simulink model "Control_v8_PID_LLSat"  (R2023b)
settings: Solver=FixedStepAuto  StartTime=0.0  StopTime=t_sim  FixedStep=TimeStep  RelTol=1e-3
values from neighbouring files (symbols this model uses):
  MODE = 2    [main_SCA_v3.m]    (also in main_SCA_v3_alt.m; main_SCA_v4_LQR.m; main_SCA_v5.m = 1)
  Use_IGRF = 0    [main_SCA.m]    (also in main_SCA_v3.m; main_SCA_v3_alt.m; main_SCA_v4_LQR.m; main_SCA_v5.m = 1)
undefined symbols (not defined in the file or in its folder): att, B, date, deg, DipoleMod, DiscIntNeverNeededParam, LLSataero, orbit, rad, s, sat
libraries: vrlib x21, aerolibutil x17, dspmathops x15, aerolibconvert2 x14, sharedtransform x14, sharedutil x5, simulink x4, simulink_extras x2, dspstat3 x1, aerolibatmos2 x1, aerolibobsolete x1
(part 2 of 3)

== system Control_v8_PID_LLSat/Attitude Reference/Switch Case Action Subsystem1 ==
  Q_retro : Inport
  W_retro : Inport  Port=2
  Action Port : ActionPort  ActionPortLabel=case [ 5 ]:
  Out1 : Outport  VectorParamsAs1DForOutWhenUnconnected=off
  Out3 : Outport  Port=2  VectorParamsAs1DForOutWhenUnconnected=off
  wires:
  Q_retro/1 -> Out1/1
  W_retro/1 -> Out3/1

== system Control_v8_PID_LLSat/Attitude Reference/Switch Case Action Subsystem10 ==
  note: from I to SS
  Q_roll : Inport
  W_roll : Inport  Port=2
  Action Port : ActionPort  ActionPortLabel=case [ 10 ]:
  Out1 : Outport  VectorParamsAs1DForOutWhenUnconnected=off
  Out3 : Outport  Port=2  VectorParamsAs1DForOutWhenUnconnected=off
  wires:
  Q_roll/1 -> Out1/1
  W_roll/1 -> Out3/1

== system Control_v8_PID_LLSat/Attitude Reference/Switch Case Action Subsystem11 ==
  note: from I to SS
  Q_roll : Inport
  W_roll : Inport  Port=2
  Action Port : ActionPort  ActionPortLabel=case [ 11 ]:
  Out1 : Outport  VectorParamsAs1DForOutWhenUnconnected=off
  Out3 : Outport  Port=2  VectorParamsAs1DForOutWhenUnconnected=off
  wires:
  Q_roll/1 -> Out1/1
  W_roll/1 -> Out3/1

== system Control_v8_PID_LLSat/Attitude Reference/Switch Case Action Subsystem2 ==
  note: q from I to O + rotation
  Q_drag : Inport
  W_drag : Inport  Port=2
  Action Port : ActionPort  ActionPortLabel=case [ 4 ]:
  Out1 : Outport  VectorParamsAs1DForOutWhenUnconnected=off
  W : Outport  Port=2
  wires:
  Q_drag/1 -> Out1/1
  W_drag/1 -> W/1

== system Control_v8_PID_LLSat/Attitude Reference/Switch Case Action Subsystem3 ==
  Q_sun_sun : Inport
  W_sun_sun : Inport  Port=2
  Action Port : ActionPort  ActionPortLabel=case [ 3 ]:
  Out1 : Outport  VectorParamsAs1DForOutWhenUnconnected=off
  Out3 : Outport  Port=2  VectorParamsAs1DForOutWhenUnconnected=off
  wires:
  Q_sun_sun/1 -> Out1/1
  W_sun_sun/1 -> Out3/1

== system Control_v8_PID_LLSat/Attitude Reference/Switch Case Action Subsystem4 ==
  Q_sun_aero : Inport
  W_sun_aero : Inport  Port=2
  Action Port : ActionPort  ActionPortLabel=case [ 2 ]:
  Out1 : Outport  VectorParamsAs1DForOutWhenUnconnected=off
  Out3 : Outport  Port=2  VectorParamsAs1DForOutWhenUnconnected=off
  wires:
  Q_sun_aero/1 -> Out1/1
  W_sun_aero/1 -> Out3/1

== system Control_v8_PID_LLSat/Attitude Reference/Switch Case Action Subsystem5 ==
  In1 : Inport
  W_orbit : Inport  Port=2
  Action Port : ActionPort  ActionPortLabel=case [ 1 ]:
  Out1 : Outport  VectorParamsAs1DForOutWhenUnconnected=off
  Out3 : Outport  Port=2  VectorParamsAs1DForOutWhenUnconnected=off
  wires:
  In1/1 -> Out1/1
  W_orbit/1 -> Out3/1

== system Control_v8_PID_LLSat/Attitude Reference/Switch Case Action Subsystem6 ==
  In1 : Inport
  In2 : Inport  Port=2
  Action Port : ActionPort  ActionPortLabel=case [ 7 ]:
  Derivative : Derivative
  Matrix Multiply : Product  Multiplication=Matrix(*)
  Quaternions to Direction Cosine Matrix : sharedtransform/Quaternions to  Direction Cosine Matrix  aMode=aMode
  Transpose : Math  Operator=transpose
  Transpose1 : Math  Operator=transpose
  gets vector from Skew Matrix : MATLABFcn  MATLABFcn=vec_from_skew
  Out1 : Outport  VectorParamsAs1DForOutWhenUnconnected=off
  W_custom : Outport  Port=2
  wires:
  In1/1 -> Out1/1
  In2/1 -> Quaternions to Direction Cosine Matrix/1
  Quaternions to Direction Cosine Matrix/1 -> Transpose1/1
  Matrix Multiply/1 -> gets vector from Skew Matrix/1
  Transpose/1 -> Derivative/1
  gets vector from Skew Matrix/1 -> W_custom/1
  Derivative/1 -> Matrix Multiply/1
  Transpose1/1 -> Transpose/1, Matrix Multiply/2

== system Control_v8_PID_LLSat/Attitude Reference/Switch Case Action Subsystem7 ==
  In1 : Inport
  In2 : Inport  Port=2
  Action Port : ActionPort  ActionPortLabel=case [ 6 ]:
  Out1 : Outport  VectorParamsAs1DForOutWhenUnconnected=off
  Out2 : Outport  Port=2  VectorParamsAs1DForOutWhenUnconnected=off
  wires:
  In1/1 -> Out1/1
  In2/1 -> Out2/1

== system Control_v8_PID_LLSat/Attitude Reference/Switch Case Action Subsystem8 ==
  Q_retro : Inport
  W_retro : Inport  Port=2
  Action Port : ActionPort  ActionPortLabel=case [ 8 ]:
  Out1 : Outport  VectorParamsAs1DForOutWhenUnconnected=off
  Out3 : Outport  Port=2  VectorParamsAs1DForOutWhenUnconnected=off
  wires:
  Q_retro/1 -> Out1/1
  W_retro/1 -> Out3/1

== system Control_v8_PID_LLSat/Attitude Reference/Switch Case Action Subsystem9 ==
  note: q from I to O + rotation
  Q_rot : Inport
  W_rot : Inport  Port=2
  Action Port : ActionPort  ActionPortLabel=case [ 9 ]:
  Out1 : Outport  VectorParamsAs1DForOutWhenUnconnected=off
  W : Outport  Port=2
  wires:
  Q_rot/1 -> Out1/1
  W_rot/1 -> W/1

== system Control_v8_PID_LLSat/Attitude Reference/q_drag ==
  note: x in BRF is aligned with the zenith direction
      | z in BRF (solar panels) is aligned in the direction of velocity
  note: DCM from Drag to Inertial
  note: q from D to I
  note: q from I to D
  note: To get angular velocity from Rotation matrix:
      | https://en.wikipedia.org/wiki/Angular_velocity#Angular_velocity_tensor
      | W= dA/dt * A'
      | $W=\frac{dA}{dt} {\dot} A'=\frac{dA}{dt} {\dot} A^{T}$
  <XYZ_ECI> : Inport
  <VxVyVz_ECI> : Inport  Port=2
  3x3 Cross Product : sharedutil/3x3 Cross Product  aMode=aMode
  Derivative : Derivative
  Direction Cosine Matrix to Quaternions : sharedtransform/Direction Cosine Matrix  to Quaternions  aMode=0  action=None  tolerance=eps(2)
  Gain : Gain
  Gain1 : Gain
  Matrix Multiply : Product  Multiplication=Matrix(*)
  Normalization : dspmathops/Normalization  NormType=2-norm  Bias=1e-10  NormOver=Each column  Dimension=1  roundingMode=Floor  overflowMode=off  accumDataTypeStr=Inherit: Same as product output  accumLastDataTypeStr=Inherit: Same as product output  outputDataTypeStr=Inherit: Same as product output  outputMin=[]  outputMax=[]  outputLastDataTypeStr=Inherit: Same as product output
  Normalization1 : dspmathops/Normalization  NormType=2-norm  Bias=1e-10  NormOver=Each column  Dimension=1  roundingMode=Floor  overflowMode=off  accumDataTypeStr=Inherit: Same as product output  accumLastDataTypeStr=Inherit: Same as product output  outputDataTypeStr=Inherit: Same as product output  outputMin=[]  outputMax=[]  outputLastDataTypeStr=Inherit: Same as product output
  Quaternion Inverse : aerolibutil/Quaternion Inverse
  Reshape : Reshape  OutputDimensionality=Column vector (2-D)
  Reshape1 : Reshape  OutputDimensionality=Column vector (2-D)
  Reshape2 : Reshape  OutputDimensionality=Column vector (2-D)
  Reshape3 : Reshape  OutputDimensionality=Customize  OutputDimensions=[3,3]
  Transpose : Math  Operator=transpose
  Vector Concatenate : Concatenate  NumInputs=3  Mode=Multidimensional array  ConcatenateDimension=2
  gets vector from Skew Matrix : MATLABFcn  MATLABFcn=vec_from_skew
  Q_drag : Outport  VectorParamsAs1DForOutWhenUnconnected=off
  W_drag : Outport  Port=2
  wires:
  Normalization/1 -> Reshape/1
  Normalization1/1 -> Reshape1/1
  <VxVyVz_ECI>/1 -> Normalization1/1
  Reshape1/1 -> Vector Concatenate/3, 3x3 Cross Product/1
  <XYZ_ECI>/1 -> Normalization/1
  Reshape/1 -> Gain/1
  Gain/1 -> Vector Concatenate/1, 3x3 Cross Product/2
  Direction Cosine Matrix to Quaternions/1 -> Quaternion Inverse/1
  3x3 Cross Product/1 -> Gain1/1
  Gain1/1 -> Reshape2/1
  Quaternion Inverse/1 -> Q_drag/1
  Vector Concatenate/1 -> Reshape3/1, Direction Cosine Matrix to Quaternions/1
  gets vector from Skew Matrix/1 -> W_drag/1
  Matrix Multiply/1 -> gets vector from Skew Matrix/1
  Transpose/1 -> Derivative/1
  Derivative/1 -> Matrix Multiply/1
  Reshape2/1 -> Vector Concatenate/2
  Reshape3/1 -> Matrix Multiply/2, Transpose/1

== system Control_v8_PID_LLSat/Attitude Reference/q_orbital ==
  note: DCM from Orbital to Inertial
  note: q from O to I
  note: q from I to O
  note: To get angular velocity from Rotation matrix:
      | https://en.wikipedia.org/wiki/Angular_velocity#Angular_velocity_tensor
      | W= dA/dt * A'
      | $W=\frac{dA}{dt} {\dot} A'=\frac{dA}{dt} {\dot} A^{T}$
  <XYZ_ECI> : Inport
  <VxVyVz_ECI> : Inport  Port=2
  3x3 Cross Product : sharedutil/3x3 Cross Product  aMode=aMode
  Derivative : Derivative
  Direction Cosine Matrix to Quaternions : sharedtransform/Direction Cosine Matrix  to Quaternions  aMode=0  action=None  tolerance=eps(2)
  Gain : Gain
  Gain1 : Gain  Gain=-1
  Matrix Multiply : Product  Multiplication=Matrix(*)
  Normalization : dspmathops/Normalization  NormType=2-norm  Bias=1e-10  NormOver=Each column  Dimension=1  roundingMode=Floor  overflowMode=off  accumDataTypeStr=Inherit: Same as product output  accumLastDataTypeStr=Inherit: Same as product output  outputDataTypeStr=Inherit: Same as product output  outputMin=[]  outputMax=[]  outputLastDataTypeStr=Inherit: Same as product output
  Normalization1 : dspmathops/Normalization  NormType=2-norm  Bias=1e-10  NormOver=Each column  Dimension=1  roundingMode=Floor  overflowMode=off  accumDataTypeStr=Inherit: Same as product output  accumLastDataTypeStr=Inherit: Same as product output  outputDataTypeStr=Inherit: Same as product output  outputMin=[]  outputMax=[]  outputLastDataTypeStr=Inherit: Same as product output
  Quaternion Inverse : aerolibutil/Quaternion Inverse
  Reshape : Reshape  OutputDimensionality=Column vector (2-D)
  Reshape1 : Reshape  OutputDimensionality=Column vector (2-D)
  Reshape2 : Reshape  OutputDimensionality=Column vector (2-D)
  Reshape3 : Reshape  OutputDimensionality=Customize  OutputDimensions=[3,3]
  Transpose : Math  Operator=transpose
  Vector Concatenate : Concatenate  NumInputs=3  Mode=Multidimensional array  ConcatenateDimension=2
  gets vector from Skew Matrix : MATLABFcn  MATLABFcn=vec_from_skew
  Q_orbit : Outport  VectorParamsAs1DForOutWhenUnconnected=off
  W_orbit : Outport  Port=2
  wires:
  Normalization/1 -> Reshape/1
  Normalization1/1 -> Reshape1/1
  <VxVyVz_ECI>/1 -> Normalization1/1
  Reshape1/1 -> 3x3 Cross Product/1, Vector Concatenate/1
  <XYZ_ECI>/1 -> Normalization/1
  Reshape/1 -> Gain/1
  Gain/1 -> 3x3 Cross Product/2, Vector Concatenate/3
  Direction Cosine Matrix to Quaternions/1 -> Quaternion Inverse/1
  3x3 Cross Product/1 -> Gain1/1
  Gain1/1 -> Reshape2/1
  Quaternion Inverse/1 -> Q_orbit/1
  Vector Concatenate/1 -> Reshape3/1, Direction Cosine Matrix to Quaternions/1
  gets vector from Skew Matrix/1 -> W_orbit/1
  Matrix Multiply/1 -> gets vector from Skew Matrix/1
  Transpose/1 -> Derivative/1
  Derivative/1 -> Matrix Multiply/1
  Reshape2/1 -> Vector Concatenate/2
  Reshape3/1 -> Matrix Multiply/2, Transpose/1

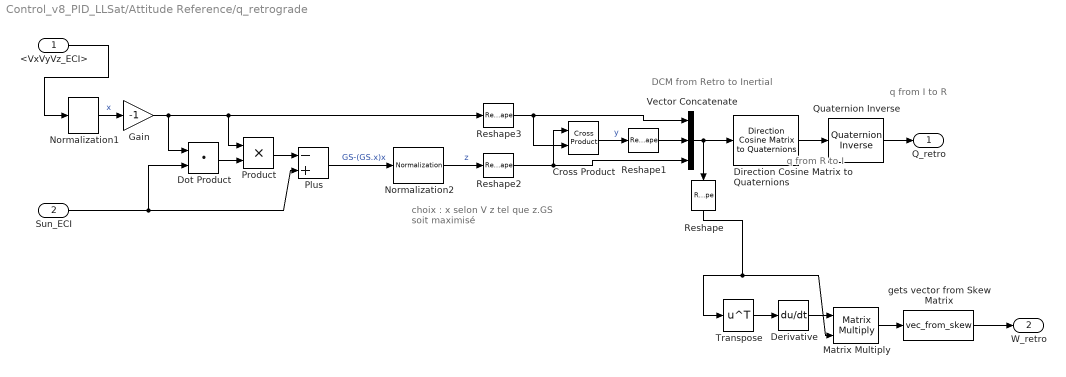
== system Control_v8_PID_LLSat/Attitude Reference/q_retrograde ==
  note: q from I to R
  note: q from R to I
  note: DCM from Retro to Inertial
  note: choix :
      | x selon V
      | z tel que z.GS soit maximisé
  <VxVyVz_ECI> : Inport
  Sun_ECI : Inport  Port=2
  Cross Product : vrlib/Utilities/Cross Product
  Derivative : Derivative
  Direction Cosine Matrix to Quaternions : sharedtransform/Direction Cosine Matrix  to Quaternions  aMode=0  action=None  tolerance=eps(2)
  Dot Product : DotProduct  OutDataTypeStr=Inherit: Inherit via internal rule
  Gain : Gain  Gain=-1
  Matrix Multiply : Product  Multiplication=Matrix(*)
  Normalization1 : dspmathops/Normalization  NormType=2-norm  Bias=1e-10  NormOver=Each column  Dimension=1  roundingMode=Floor  overflowMode=off  accumDataTypeStr=Inherit: Same as product output  accumLastDataTypeStr=Inherit: Same as product output  outputDataTypeStr=Inherit: Same as product output  outputMin=[]  outputMax=[]  outputLastDataTypeStr=Inherit: Same as product output
  Normalization2 : dspmathops/Normalization  NormType=2-norm  Bias=1e-10  NormOver=Each column  Dimension=1  roundingMode=Floor  overflowMode=off  accumDataTypeStr=Inherit: Same as product output  accumLastDataTypeStr=Inherit: Same as product output  outputDataTypeStr=Inherit: Same as product output  outputMin=[]  outputMax=[]  outputLastDataTypeStr=Inherit: Same as product output
  Plus : Sum  Inputs=-+
  Product : Product
  Quaternion Inverse : aerolibutil/Quaternion Inverse
  Reshape : Reshape  OutputDimensionality=Customize  OutputDimensions=[3,3]
  Reshape1 : Reshape  OutputDimensionality=Column vector (2-D)
  Reshape2 : Reshape  OutputDimensionality=Column vector (2-D)
  Reshape3 : Reshape  OutputDimensionality=Column vector (2-D)
  Transpose : Math  Operator=transpose
  Vector Concatenate : Concatenate  NumInputs=3  Mode=Multidimensional array  ConcatenateDimension=2
  gets vector from Skew Matrix : MATLABFcn  MATLABFcn=vec_from_skew
  Q_retro : Outport  VectorParamsAs1DForOutWhenUnconnected=off
  W_retro : Outport  Port=2
  wires:
  Quaternion Inverse/1 -> Q_retro/1
  Reshape2/1 -> Vector Concatenate/3, Cross Product/1
  Reshape3/1 -> Vector Concatenate/1, Cross Product/2
  Product/1 -> Plus/1
  Dot Product/1 -> Product/2
  Cross Product/1 -> Reshape1/1  "y"
  Normalization2/1 -> Reshape2/1  "z"
  Plus/1 -> Normalization2/1  "GS-(GS.x)x"
  Sun_ECI/1 -> Dot Product/2, Plus/2
  Direction Cosine Matrix to Quaternions/1 -> Quaternion Inverse/1
  Normalization1/1 -> Gain/1  "x"
  <VxVyVz_ECI>/1 -> Normalization1/1
  Reshape1/1 -> Vector Concatenate/2
  Gain/1 -> Dot Product/1, Product/1, Reshape3/1
  Vector Concatenate/1 -> Direction Cosine Matrix to Quaternions/1, Reshape/1
  gets vector from Skew Matrix/1 -> W_retro/1
  Matrix Multiply/1 -> gets vector from Skew Matrix/1
  Derivative/1 -> Matrix Multiply/1
  Transpose/1 -> Derivative/1
  Reshape/1 -> Transpose/1, Matrix Multiply/2

== system Control_v8_PID_LLSat/Attitude Reference/q_sun_aero ==
  note: q from I to S
  note: q from S to I
  note: DCM from Sun-aero to Inertial
  note: choix :
      | x selon V
      | z tel que z.GS soit maximisé
  Sun_ECI : Inport
  <VxVyVz_ECI> : Inport  Port=2
  Cross Product : vrlib/Utilities/Cross Product
  Derivative : Derivative
  Direction Cosine Matrix to Quaternions : sharedtransform/Direction Cosine Matrix  to Quaternions  aMode=0  action=None  tolerance=eps(2)
  Dot Product : DotProduct  OutDataTypeStr=Inherit: Inherit via internal rule
  Matrix Multiply : Product  Multiplication=Matrix(*)
  Normalization1 : dspmathops/Normalization  NormType=2-norm  Bias=1e-10  NormOver=Each column  Dimension=1  roundingMode=Floor  overflowMode=off  accumDataTypeStr=Inherit: Same as product output  accumLastDataTypeStr=Inherit: Same as product output  outputDataTypeStr=Inherit: Same as product output  outputMin=[]  outputMax=[]  outputLastDataTypeStr=Inherit: Same as product output
  Normalization2 : dspmathops/Normalization  NormType=2-norm  Bias=1e-10  NormOver=Each column  Dimension=1  roundingMode=Floor  overflowMode=off  accumDataTypeStr=Inherit: Same as product output  accumLastDataTypeStr=Inherit: Same as product output  outputDataTypeStr=Inherit: Same as product output  outputMin=[]  outputMax=[]  outputLastDataTypeStr=Inherit: Same as product output
  Plus : Sum  Inputs=-+
  Product : Product
  Quaternion Inverse : aerolibutil/Quaternion Inverse
  Reshape : Reshape  OutputDimensionality=Customize  OutputDimensions=[3,3]
  Reshape1 : Reshape  OutputDimensionality=Column vector (2-D)
  Reshape2 : Reshape  OutputDimensionality=Column vector (2-D)
  Reshape3 : Reshape  OutputDimensionality=Column vector (2-D)
  Transpose : Math  Operator=transpose
  Vector Concatenate : Concatenate  NumInputs=3  Mode=Multidimensional array  ConcatenateDimension=2
  gets vector from Skew Matrix : MATLABFcn  MATLABFcn=vec_from_skew
  Q_sun_aero : Outport  VectorParamsAs1DForOutWhenUnconnected=off
  W_sun_aero : Outport  Port=2
  wires:
  Quaternion Inverse/1 -> Q_sun_aero/1
  Reshape2/1 -> Vector Concatenate/3, Cross Product/1
  Reshape3/1 -> Vector Concatenate/1, Cross Product/2
  Product/1 -> Plus/1
  Dot Product/1 -> Product/2
  Cross Product/1 -> Reshape1/1  "y"
  Normalization2/1 -> Reshape2/1  "z"
  Plus/1 -> Normalization2/1  "GS-(GS.x)x"
  Sun_ECI/1 -> Dot Product/2, Plus/2
  Direction Cosine Matrix to Quaternions/1 -> Quaternion Inverse/1
  Normalization1/1 -> Dot Product/1, Product/1, Reshape3/1  "x"
  <VxVyVz_ECI>/1 -> Normalization1/1
  Reshape1/1 -> Vector Concatenate/2
  Transpose/1 -> Derivative/1
  Matrix Multiply/1 -> gets vector from Skew Matrix/1
  Derivative/1 -> Matrix Multiply/1
  Vector Concatenate/1 -> Direction Cosine Matrix to Quaternions/1, Reshape/1
  gets vector from Skew Matrix/1 -> W_sun_aero/1
  Reshape/1 -> Transpose/1, Matrix Multiply/2

== system Control_v8_PID_LLSat/Attitude Reference/q_sun_aero_rotation_x_pi//1 ==
  Q_sun_aero : Inport
  Q_sun_sun : Inport  Port=2
  In3 : Inport  Port=3
  Quaternion Interpolation : QuatInterp
  Quaternion Normalize : sharedutil/Quaternion Normalize  aMode=aMode
  Quaternion Normalize1 : sharedutil/Quaternion Normalize  aMode=aMode
  Q_slerp : Outport  VectorParamsAs1DForOutWhenUnconnected=off
  wires:
  Quaternion Interpolation/1 -> Q_slerp/1
  Q_sun_sun/1 -> Quaternion Normalize1/1
  Q_sun_aero/1 -> Quaternion Normalize/1
  In3/1 -> Quaternion Interpolation/3
  Quaternion Normalize/1 -> Quaternion Interpolation/1
  Quaternion Normalize1/1 -> Quaternion Interpolation/2

== system Control_v8_PID_LLSat/Attitude Reference/q_sun_aero_rotation_x_pi//4 ==
  Constant : Constant  Value=[1;0;0]
  Product : Product
  Reshape1 : Reshape  OutputDimensionality=Column vector (2-D)
  Vector Concatenate1 : Concatenate  Mode=Multidimensional array
  cos pi/2 : Constant  Value=[cos(-att.angle_roll/2)]
  sin pi/4 : Constant  Value=sin(-att.angle_roll/2)
  Q_rot : Outport  VectorParamsAs1DForOutWhenUnconnected=off
  wires:
  cos pi/2/1 -> Vector Concatenate1/1
  Vector Concatenate1/1 -> Q_rot/1
  sin pi/4/1 -> Product/2
  Product/1 -> Reshape1/1
  Reshape1/1 -> Vector Concatenate1/2
  Constant/1 -> Product/1  "x"

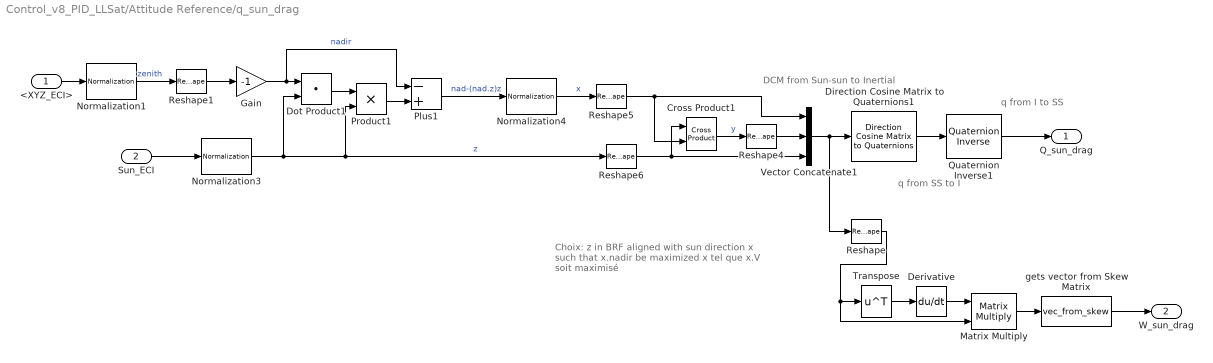
== system Control_v8_PID_LLSat/Attitude Reference/q_sun_drag ==
  note: Choix:
      | z in BRF aligned with sun direction
      | x such that x.nadir be maximized
      | x tel que x.V soit maximisé
  note: DCM from Sun-sun to Inertial
  note: q from I to SS
  note: q from SS to I
  <XYZ_ECI> : Inport
  Sun_ECI : Inport  Port=2
  Cross Product1 : vrlib/Utilities/Cross Product
  Derivative : Derivative
  Direction Cosine Matrix to Quaternions1 : sharedtransform/Direction Cosine Matrix  to Quaternions  aMode=0  action=None  tolerance=eps(2)
  Dot Product1 : DotProduct  OutDataTypeStr=Inherit: Inherit via internal rule
  Gain : Gain  Gain=-1
  Matrix Multiply : Product  Multiplication=Matrix(*)
  Normalization1 : dspmathops/Normalization  NormType=2-norm  Bias=1e-10  NormOver=Each column  Dimension=1  roundingMode=Floor  overflowMode=off  accumDataTypeStr=Inherit: Same as product output  accumLastDataTypeStr=Inherit: Same as product output  outputDataTypeStr=Inherit: Same as product output  outputMin=[]  outputMax=[]  outputLastDataTypeStr=Inherit: Same as product output
  Normalization3 : dspmathops/Normalization  NormType=2-norm  Bias=1e-10  NormOver=Each column  Dimension=1  roundingMode=Floor  overflowMode=off  accumDataTypeStr=Inherit: Same as product output  accumLastDataTypeStr=Inherit: Same as product output  outputDataTypeStr=Inherit: Same as product output  outputMin=[]  outputMax=[]  outputLastDataTypeStr=Inherit: Same as product output
  Normalization4 : dspmathops/Normalization  NormType=2-norm  Bias=1e-10  NormOver=Each column  Dimension=1  roundingMode=Floor  overflowMode=off  accumDataTypeStr=Inherit: Same as product output  accumLastDataTypeStr=Inherit: Same as product output  outputDataTypeStr=Inherit: Same as product output  outputMin=[]  outputMax=[]  outputLastDataTypeStr=Inherit: Same as product output
  Plus1 : Sum  Inputs=-+
  Product1 : Product
  Quaternion Inverse1 : aerolibutil/Quaternion Inverse
  Reshape : Reshape  OutputDimensionality=Customize  OutputDimensions=[3,3]
  Reshape{1,4..6} (4 alike) : Reshape  OutputDimensionality=Column vector (2-D)
  Transpose : Math  Operator=transpose
  Vector Concatenate1 : Concatenate  NumInputs=3  Mode=Multidimensional array  ConcatenateDimension=2
  gets vector from Skew Matrix : MATLABFcn  MATLABFcn=vec_from_skew
  Q_sun_drag : Outport  VectorParamsAs1DForOutWhenUnconnected=off
  W_sun_drag : Outport  Port=2
  wires:
  Direction Cosine Matrix to Quaternions1/1 -> Quaternion Inverse1/1
  Reshape4/1 -> Vector Concatenate1/2
  Dot Product1/1 -> Product1/1
  Sun_ECI/1 -> Normalization3/1
  Quaternion Inverse1/1 -> Q_sun_drag/1
  Reshape1/1 -> Gain/1
  Plus1/1 -> Normalization4/1  "nad-(nad.z)z"
  Reshape6/1 -> Cross Product1/1, Vector Concatenate1/3
  Normalization3/1 -> Dot Product1/2, Product1/2, Reshape6/1  "z"
  Reshape5/1 -> Cross Product1/2, Vector Concatenate1/1
  Cross Product1/1 -> Reshape4/1  "y"
  Normalization4/1 -> Reshape5/1  "x"
  Product1/1 -> Plus1/2
  Reshape/1 -> Matrix Multiply/2, Transpose/1
  Derivative/1 -> Matrix Multiply/1
  Transpose/1 -> Derivative/1
  Matrix Multiply/1 -> gets vector from Skew Matrix/1
  gets vector from Skew Matrix/1 -> W_sun_drag/1
  Vector Concatenate1/1 -> Direction Cosine Matrix to Quaternions1/1, Reshape/1
  <XYZ_ECI>/1 -> Normalization1/1
  Normalization1/1 -> Reshape1/1  "zenith"
  Gain/1 -> Dot Product1/1, Plus1/1  "nadir"

== system Control_v8_PID_LLSat/Attitude Reference/q_sun_sun ==
  note: Choix:
      | z selon GS
      | x tel que x.V soit maximisé
  note: DCM from Sun-sun to Inertial
  note: q from I to SS
  note: q from SS to I
  <VxVyVz_ECI> : Inport
  Sun_ECI : Inport  Port=2
  Cross Product1 : vrlib/Utilities/Cross Product
  Derivative : Derivative
  Direction Cosine Matrix to Quaternions1 : sharedtransform/Direction Cosine Matrix  to Quaternions  aMode=0  action=None  tolerance=eps(2)
  Dot Product1 : DotProduct  OutDataTypeStr=Inherit: Inherit via internal rule
  Matrix Multiply : Product  Multiplication=Matrix(*)
  Normalization3 : dspmathops/Normalization  NormType=2-norm  Bias=1e-10  NormOver=Each column  Dimension=1  roundingMode=Floor  overflowMode=off  accumDataTypeStr=Inherit: Same as product output  accumLastDataTypeStr=Inherit: Same as product output  outputDataTypeStr=Inherit: Same as product output  outputMin=[]  outputMax=[]  outputLastDataTypeStr=Inherit: Same as product output
  Normalization4 : dspmathops/Normalization  NormType=2-norm  Bias=1e-10  NormOver=Each column  Dimension=1  roundingMode=Floor  overflowMode=off  accumDataTypeStr=Inherit: Same as product output  accumLastDataTypeStr=Inherit: Same as product output  outputDataTypeStr=Inherit: Same as product output  outputMin=[]  outputMax=[]  outputLastDataTypeStr=Inherit: Same as product output
  Plus1 : Sum  Inputs=-+
  Product1 : Product
  Quaternion Inverse1 : aerolibutil/Quaternion Inverse
  Reshape : Reshape  OutputDimensionality=Customize  OutputDimensions=[3,3]
  Reshape4 : Reshape  OutputDimensionality=Column vector (2-D)
  Reshape5 : Reshape  OutputDimensionality=Column vector (2-D)
  Reshape6 : Reshape  OutputDimensionality=Column vector (2-D)
  Transpose : Math  Operator=transpose
  Vector Concatenate1 : Concatenate  NumInputs=3  Mode=Multidimensional array  ConcatenateDimension=2
  gets vector from Skew Matrix : MATLABFcn  MATLABFcn=vec_from_skew
  Q_sun_sun : Outport  VectorParamsAs1DForOutWhenUnconnected=off
  W_sun_sun : Outport  Port=2
  wires:
  Direction Cosine Matrix to Quaternions1/1 -> Quaternion Inverse1/1
  Reshape4/1 -> Vector Concatenate1/2
  Dot Product1/1 -> Product1/1
  Sun_ECI/1 -> Normalization3/1
  Quaternion Inverse1/1 -> Q_sun_sun/1
  <VxVyVz_ECI>/1 -> Dot Product1/1, Plus1/1
  Plus1/1 -> Normalization4/1  "V-(V.z)z"
  Reshape6/1 -> Cross Product1/1, Vector Concatenate1/3
  Normalization3/1 -> Dot Product1/2, Product1/2, Reshape6/1  "z"
  Reshape5/1 -> Cross Product1/2, Vector Concatenate1/1
  Cross Product1/1 -> Reshape4/1  "y"
  Normalization4/1 -> Reshape5/1  "x"
  Product1/1 -> Plus1/2
  Reshape/1 -> Matrix Multiply/2, Transpose/1
  Derivative/1 -> Matrix Multiply/1
  Transpose/1 -> Derivative/1
  Matrix Multiply/1 -> gets vector from Skew Matrix/1
  gets vector from Skew Matrix/1 -> W_sun_sun/1
  Vector Concatenate1/1 -> Direction Cosine Matrix to Quaternions1/1, Reshape/1

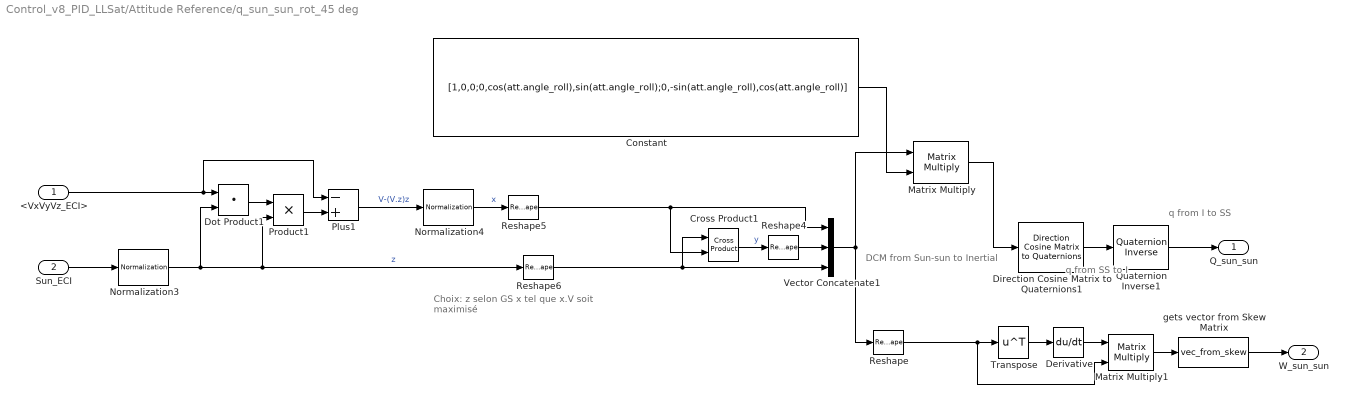
== system Control_v8_PID_LLSat/Attitude Reference/q_sun_sun_rot_45 deg ==
  note: Choix:
      | z selon GS
      | x tel que x.V soit maximisé
  note: DCM from Sun-sun to Inertial
  note: q from I to SS
  note: q from SS to I
  <VxVyVz_ECI> : Inport
  Sun_ECI : Inport  Port=2
  Constant : Constant  Value=[1,0,0;0,cos(att.angle_roll),sin(att.angle_roll);0,-sin(att.angle_roll),cos(att.angle_roll)]
  Cross Product1 : vrlib/Utilities/Cross Product
  Derivative : Derivative
  Direction Cosine Matrix to Quaternions1 : sharedtransform/Direction Cosine Matrix  to Quaternions  aMode=0  action=None  tolerance=eps(2)
  Dot Product1 : DotProduct  OutDataTypeStr=Inherit: Inherit via internal rule
  Matrix Multiply : Product  Multiplication=Matrix(*)
  Matrix Multiply1 : Product  Multiplication=Matrix(*)
  Normalization3 : dspmathops/Normalization  NormType=2-norm  Bias=1e-10  NormOver=Each column  Dimension=1  roundingMode=Floor  overflowMode=off  accumDataTypeStr=Inherit: Same as product output  accumLastDataTypeStr=Inherit: Same as product output  outputDataTypeStr=Inherit: Same as product output  outputMin=[]  outputMax=[]  outputLastDataTypeStr=Inherit: Same as product output
  Normalization4 : dspmathops/Normalization  NormType=2-norm  Bias=1e-10  NormOver=Each column  Dimension=1  roundingMode=Floor  overflowMode=off  accumDataTypeStr=Inherit: Same as product output  accumLastDataTypeStr=Inherit: Same as product output  outputDataTypeStr=Inherit: Same as product output  outputMin=[]  outputMax=[]  outputLastDataTypeStr=Inherit: Same as product output
  Plus1 : Sum  Inputs=-+
  Product1 : Product
  Quaternion Inverse1 : aerolibutil/Quaternion Inverse
  Reshape : Reshape  OutputDimensionality=Customize  OutputDimensions=[3,3]
  Reshape4 : Reshape  OutputDimensionality=Column vector (2-D)
  Reshape5 : Reshape  OutputDimensionality=Column vector (2-D)
  Reshape6 : Reshape  OutputDimensionality=Column vector (2-D)
  Transpose : Math  Operator=transpose
  Vector Concatenate1 : Concatenate  NumInputs=3  Mode=Multidimensional array  ConcatenateDimension=2
  gets vector from Skew Matrix : MATLABFcn  MATLABFcn=vec_from_skew
  Q_sun_sun : Outport  VectorParamsAs1DForOutWhenUnconnected=off
  W_sun_sun : Outport  Port=2
  wires:
  Reshape4/1 -> Vector Concatenate1/2
  Dot Product1/1 -> Product1/1
  Sun_ECI/1 -> Normalization3/1
  Quaternion Inverse1/1 -> Q_sun_sun/1
  <VxVyVz_ECI>/1 -> Dot Product1/1, Plus1/1
  Plus1/1 -> Normalization4/1  "V-(V.z)z"
  Reshape6/1 -> Cross Product1/1, Vector Concatenate1/3
  Normalization3/1 -> Dot Product1/2, Product1/2, Reshape6/1  "z"
  Reshape5/1 -> Cross Product1/2, Vector Concatenate1/1
  Cross Product1/1 -> Reshape4/1  "y"
  Normalization4/1 -> Reshape5/1  "x"
  Product1/1 -> Plus1/2
  Direction Cosine Matrix to Quaternions1/1 -> Quaternion Inverse1/1
  Constant/1 -> Matrix Multiply/2
  Vector Concatenate1/1 -> Matrix Multiply/1, Reshape/1
  Matrix Multiply/1 -> Direction Cosine Matrix to Quaternions1/1
  Transpose/1 -> Derivative/1
  gets vector from Skew Matrix/1 -> W_sun_sun/1
  Reshape/1 -> Matrix Multiply1/2, Transpose/1
  Derivative/1 -> Matrix Multiply1/1
  Matrix Multiply1/1 -> gets vector from Skew Matrix/1

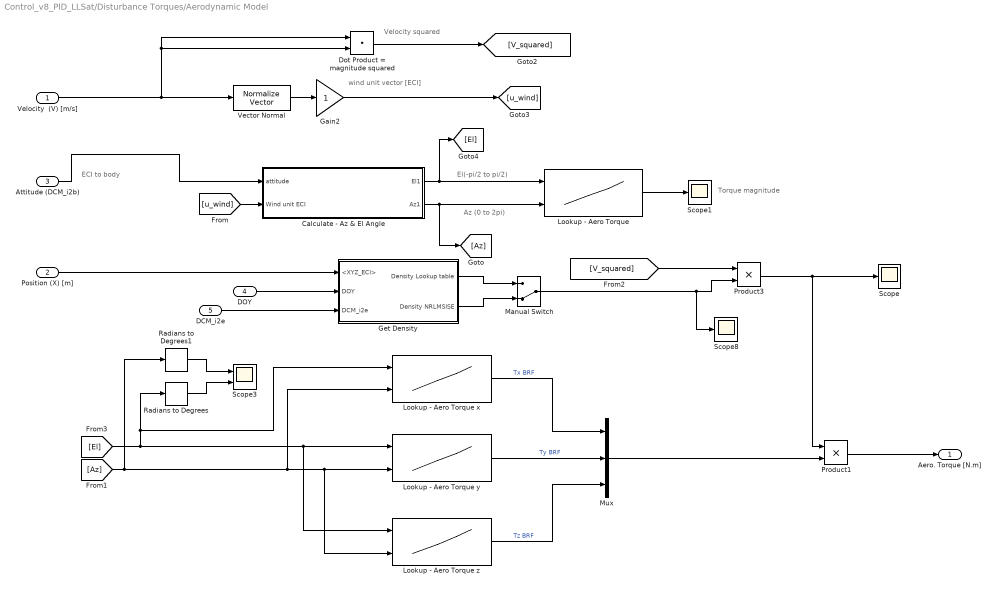
== system Control_v8_PID_LLSat/Disturbance Torques/Aerodynamic Model ==
  note: Az (0 to 2pi)
  note: wind unit vector [ECI]
  note: Torque magnitude
  note: ECI to body
  note: Velocity squared
  note: El(-pi/2 to pi/2)
  Velocity  (V) [m/s] : Inport
  Position (X) [m] : Inport  Port=2
  Attitude (DCM_i2b) : Inport  Port=3
  DOY : Inport  Port=4
  DCM_i2e : Inport  Port=5
  Calculate - Az & El Angle : Subsystem
  Dot Product = magnitude squared : DotProduct  OutDataTypeStr=Inherit: Inherit via internal rule
  Gain2 : Gain
  Get Density : Subsystem
  Lookup - Aero Torque : Lookup2D  RowIndex=LLSataero.Az  ColumnIndex=LLSataero.El  Table=LLSataero.T  SaturateOnIntegerOverflow=off  InputSameDT=off
  Lookup - Aero Torque x : Lookup2D  RowIndex=LLSataero.Az  ColumnIndex=LLSataero.El  Table=LLSataero.Tx  SaturateOnIntegerOverflow=off  InputSameDT=off
  Lookup - Aero Torque y : Lookup2D  RowIndex=LLSataero.Az  ColumnIndex=LLSataero.El  Table=LLSataero.Ty  SaturateOnIntegerOverflow=off  InputSameDT=off
  Lookup - Aero Torque z : Lookup2D  RowIndex=LLSataero.Az  ColumnIndex=LLSataero.El  Table=LLSataero.Tz  SaturateOnIntegerOverflow=off  InputSameDT=off
  Manual Switch : ManualSwitch  CurrentSetting=0
  Mux : Mux  Inputs=3
  Product1 : Product  RndMeth=Zero
  Product3 : Product  RndMeth=Zero
  Radians to Degrees : simulink_extras/Transformations/Radians to Degrees
  Radians to Degrees1 : simulink_extras/Transformations/Radians to Degrees
  Scope : Scope
  Scope1 : Scope
  Scope3 : Scope  NumInputPorts=2
  Scope8 : Scope
  Vector Normal : vrlib/Utilities/Normalize Vector  maxzero=0
  Aero. Torque [N.m] : Outport
  wires:
  Dot Product = magnitude squared/1 -> [V_squared]
  Vector Normal/1 -> Gain2/1
  Gain2/1 -> [u_wind]
  Lookup - Aero Torque/1 -> Scope1/1
  Attitude (DCM_i2b)/1 -> Calculate - Az & El Angle/1(attitude)
  [V_squared] -> Product3/1
  Velocity  (V) [m/s]/1 -> Dot Product = magnitude squared/2, Dot Product = magnitude squared/1, Vector Normal/1
  Radians to Degrees1/1 -> Scope3/1
  Radians to Degrees/1 -> Scope3/2
  [u_wind] -> Calculate - Az & El Angle/2(Wind unit ECI)
  Calculate - Az & El Angle/2(Az1) -> [Az], Lookup - Aero Torque/2
  Calculate - Az & El Angle/1(El1) -> [El], Lookup - Aero Torque/1
  [El] -> Lookup - Aero Torque z/1, Lookup - Aero Torque y/1, Lookup - Aero Torque x/1, Radians to Degrees/1
  [Az] -> Radians to Degrees1/1, Lookup - Aero Torque z/2, Lookup - Aero Torque y/2, Lookup - Aero Torque x/2
  Lookup - Aero Torque y/1 -> Mux/2  "Ty BRF"
  Lookup - Aero Torque x/1 -> Mux/1  "Tx BRF"
  Lookup - Aero Torque z/1 -> Mux/3  "Tz BRF"
  Mux/1 -> Product1/2
  Product3/1 -> Product1/1, Scope/1
  Product1/1 -> Aero. Torque [N.m]/1
  Manual Switch/1 -> Scope8/1, Product3/2
  Position (X) [m]/1 -> Get Density/1(<XYZ_ECI>)
  DOY/1 -> Get Density/2(DOY)
  DCM_i2e/1 -> Get Density/3("DCM_i2e ")
  Get Density/2(Density NRLMSISE) -> Manual Switch/2
  Get Density/1(Density Lookup table) -> Manual Switch/1

== system Control_v8_PID_LLSat/Disturbance Torques/Gravity Gradient Model ==
  note: \tau_{gg}= 3\mu/r^{3} (u_{nadir}\times J* u_{nadir})
  note: (3*mu/Rs^4*) * Rs = (3*mu/Rs^3) * rs
  note: Nadir [body]
  note: position of satellite [ECI]
  note: Nadir unit vector
      | [body]
  note: Anti-nadir [body]
  note: r^4
  "Position (X) [m] " : Inport
  Attitude (DCMi2b) : Inport  Port=2
  3 * mu : Constant  Value=3*3.9860044188e14
  Cross Product : vrlib/Utilities/Cross Product
  Divide : Product  Inputs=*/
  Dot Product = magnitude squared : DotProduct  OutDataTypeStr=Inherit: Inherit via internal rule
  Gain : Gain  Gain=-1
  Gain1 : Gain  Gain=-1
  J : Constant  Value=sat.inertia
  Math Function : Math  Operator=square  SignedPower=on
  Product (not cross) : Product  RndMeth=Zero
  Vector Normal : vrlib/Utilities/Normalize Vector  maxzero=0
  product 1 : Product  Multiplication=Matrix(*)  RndMeth=Zero
  product 2 : Product  Multiplication=Matrix(*)  RndMeth=Zero
  Gravity Gradient [N.m] : Outport
  wires:
  Product (not cross)/1 -> Cross Product/1
  Divide/1 -> Product (not cross)/2
  3 * mu/1 -> Divide/1
  Math Function/1 -> Divide/2
  Vector Normal/1 -> Gain/1
  Cross Product/1 -> Gravity Gradient [N.m]/1
  Dot Product = magnitude squared/1 -> Math Function/1
  Gain/1 -> product 2/2
  product 2/1 -> Cross Product/2
  J/1 -> product 2/1
  Attitude (DCMi2b)/1 -> product 1/1
  product 1/1 -> Vector Normal/1, Gain1/1
  Gain1/1 -> Product (not cross)/1
  "Position (X) [m] "/1 -> product 1/2, Dot Product = magnitude squared/2, Dot Product = magnitude squared/1

== system Control_v8_PID_LLSat/Disturbance Torques/Magnetic Torque Model ==
  note: T = m X B
  note: B_earth [body]
  note: ECI to Body
  B (ECI) : Inport
  Attitude (DCMi2b) : Inport  Port=2
  Cross Product : vrlib/Utilities/Cross Product
  Product : Product  Multiplication=Matrix(*)  RndMeth=Zero
  constant : Constant  Value=sat.residual_dipole
  MagneticTorque (N.m) : Outport
  wires:
  Product/1 -> Cross Product/2
  Cross Product/1 -> MagneticTorque (N.m)/1
  constant/1 -> Cross Product/1
  Attitude (DCMi2b)/1 -> Product/1
  B (ECI)/1 -> Product/2

== system Control_v8_PID_LLSat/IGRF Computation block/Obtain B_ECI ==
  In1 : Inport
  Dipole Subsystem : Subsystem  TreatAsAtomicUnit=on
  IGRF Subsystem : Subsystem  TreatAsAtomicUnit=on
  If : If
  Merge : Merge
  Use_IGRF : Constant  Value=Use_IGRF
  u : Outport  VectorParamsAs1DForOutWhenUnconnected=off
  wires:
  If/1 -> IGRF Subsystem/Action
  In1/1 -> Dipole Subsystem/1(In1), IGRF Subsystem/1(In1)
  IGRF Subsystem/1(Out1) -> Merge/1
  Use_IGRF/1 -> If/1
  Merge/1 -> u/1
  Dipole Subsystem/1("B_ECI ") -> Merge/2
  If/2 -> Dipole Subsystem/Action

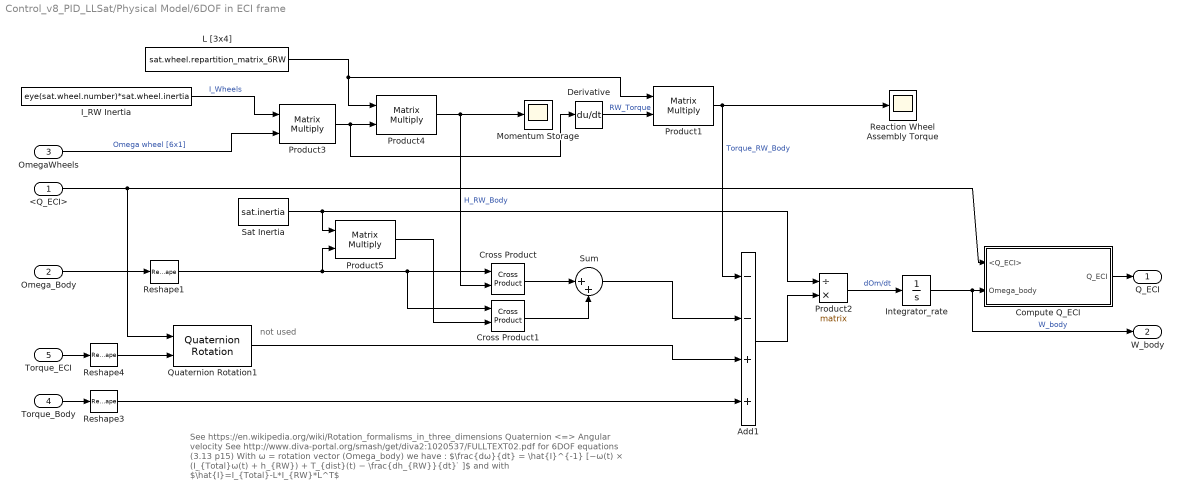
== system Control_v8_PID_LLSat/Physical Model/6DOF in ECI frame ==
  note: not used
  note: See https://en.wikipedia.org/wiki/Rotation_formalisms_in_three_dimensions Quaternion <=> Angular velocity
      |
      | See http://www.diva-portal.org/smash/get/diva2:1020537/FULLTEXT02.pdf for 6DOF equations (3.13 p15)
      |
      | With ω = rotation vector (Omega_body) we have :
      |
      | $\frac{dω}{dt} = \hat{I}^{-1} [−ω(t) × (I_{Total}ω(t) + h_{RW}) + T_{dist}(t) − \frac{dh_{RW}}{dt} ̇ ]$
      | and with $\hat{I}=I_{Total}-L*I_{RW}*L^T$
  <Q_ECI> : Inport
  "Omega_Body " : Inport  Port=2
  OmegaWheels : Inport  Port=3
  Torque_Body : Inport  Port=4
  Torque_ECI : Inport  Port=5  PortDimensions=3
  Add1 : Sum  Inputs=--++
  Compute Q_ECI : Subsystem
  Cross Product : vrlib/Utilities/Cross Product
  Cross Product1 : vrlib/Utilities/Cross Product
  Derivative : Derivative
  I_RW Inertia : Constant  Value=eye(sat.wheel.number)*sat.wheel.inertia
  Integrator_rate : Integrator
  L [3x4] : Constant  Value=sat.wheel.repartition_matrix_6RW
  Momentum Storage : Scope
  Product{1,3..5} (4 alike) : Product  Multiplication=Matrix(*)
  Product2 : Product  Inputs=/*  Multiplication=Matrix(*)
  Quaternion Rotation1 : aerolibutil/Quaternion Rotation
  Reaction Wheel Assembly Torque : Scope
  Reshape1 : Reshape  OutputDimensionality=Column vector (2-D)
  Reshape3 : Reshape  OutputDimensionality=Column vector (2-D)
  Reshape4 : Reshape  OutputDimensionality=Column vector (2-D)
  Sat Inertia : Constant  Value=sat.inertia
  Sum : Sum  Inputs=|++
  Q_ECI : Outport  VectorParamsAs1DForOutWhenUnconnected=off
  W_body : Outport  Port=2  VectorParamsAs1DForOutWhenUnconnected=off
  wires:
  Product2/1 -> Integrator_rate/1  "dOm/dt"
  Product3/1 -> Derivative/1, Product4/2
  Sat Inertia/1 -> Product5/1, Product2/1
  Add1/1 -> Product2/2
  Cross Product/1 -> Sum/1
  "Omega_Body "/1 -> Reshape1/1
  Integrator_rate/1 -> W_body/1, Compute Q_ECI/2(Omega_body)  "W_body"
  I_RW Inertia/1 -> Product3/1  "I_Wheels"
  Torque_Body/1 -> Reshape3/1
  Product1/1 -> Add1/1, Reaction Wheel Assembly Torque/1  "Torque_RW_Body"
  OmegaWheels/1 -> Product3/2  "Omega wheel [6x1]"
  Compute Q_ECI/1(Q_ECI) -> Q_ECI/1
  Torque_ECI/1 -> Reshape4/1
  <Q_ECI>/1 -> Quaternion Rotation1/1, Compute Q_ECI/1(<Q_ECI>)
  Quaternion Rotation1/1 -> Add1/3
  L [3x4]/1 -> Product1/1, Product4/1
  Reshape3/1 -> Add1/4
  Reshape4/1 -> Quaternion Rotation1/2
  Product4/1 -> Momentum Storage/1, Cross Product/2  "H_RW_Body"
  Reshape1/1 -> Product5/2, Cross Product1/1, Cross Product/1
  Derivative/1 -> Product1/2  "RW_Torque"
  Sum/1 -> Add1/2
  Cross Product1/1 -> Sum/2
  Product5/1 -> Cross Product1/2

== system Control_v8_PID_LLSat/Physical Model/Magnetorquer physics ==
  note: On pourrait aussi changer les blocs
      | magnétocoupleurs pour sortir les intensités
  Mag vector command : Inport
  B_IGRF_body (vecteur) : Inport  Port=2
  Add1 : Sum  Inputs=+++
  Cross Product : vrlib/Utilities/Cross Product
  Demux : Demux  Outputs=3
  Magnétocoupleur 1 : Subsystem
  Magnétocoupleur 2 : Subsystem
  Magnétocoupleur 3 : Subsystem
  Couple (vect) : Outport  PortDimensions=3  VectorParamsAs1DForOutWhenUnconnected=off
  Real mag moments vector : Outport  Port=2  VectorParamsAs1DForOutWhenUnconnected=off
  wires:
  Add1/1 -> Real mag moments vector/1, Cross Product/1  "M_real"
  Demux/1 -> Magnétocoupleur 1/1(m_in (scalar))
  Demux/2 -> Magnétocoupleur 2/1(m_in (scalar))
  Demux/3 -> Magnétocoupleur 3/1(m_in (scalar))
  Mag vector command/1 -> Demux/1
  Magnétocoupleur 2/1(m_out (vect)) -> Add1/2
  Magnétocoupleur 1/1(m_out (vect)) -> Add1/1
  Magnétocoupleur 3/1(m_out (vect)) -> Add1/3
  Cross Product/1 -> Couple (vect)/1  "T_body"
  B_IGRF_body (vecteur)/1 -> Cross Product/2

== system Control_v8_PID_LLSat/Physical Model/Thruster ==
  On/Off (Boolean) : Inport  OutDataTypeStr=boolean
  Constant : Constant  Value=0
  Cross Product : vrlib/Utilities/Cross Product
  If : If  IfExpression=u1
  If Action Subsystem : Subsystem  TreatAsAtomicUnit=on
  If Action Subsystem1 : Subsystem  TreatAsAtomicUnit=on
  Merge : Merge
  Product : Product
  Sum : Sum  Inputs=|-+
  Thruster Force : Constant  Value=sat.thruster.force
  unit vector of thrust : Constant  Value=sat.thruster.dir
  vector CoG : Constant  Value=sat.CoG
  vector G-Thrust point : Constant  Value=sat.thruster.point
  Force (G_sat) : Outport  VectorParamsAs1DForOutWhenUnconnected=off
  Moment (G_sat) : Outport  Port=2  VectorParamsAs1DForOutWhenUnconnected=off
  wires:
  Product/1 -> Force (G_sat)/1, Cross Product/2
  Sum/1 -> Cross Product/1
  unit vector of thrust/1 -> Product/1
  Cross Product/1 -> Moment (G_sat)/1
  Thruster Force/1 -> If Action Subsystem/1(In1)
  On/Off (Boolean)/1 -> If/1
  If/1 -> If Action Subsystem/Action
  If/2 -> If Action Subsystem1/Action
  If Action Subsystem1/1(Out1) -> Merge/2
  If Action Subsystem/1(Out1) -> Merge/1
  Merge/1 -> Product/2
  Constant/1 -> If Action Subsystem1/1(In1)
  vector G-Thrust point/1 -> Sum/1
  vector CoG/1 -> Sum/2

== system Control_v8_PID_LLSat/Attitude Controller/Magnetorquer Magnetic Momend Command/Switch Case Action Subsystem3 ==
  In1 : Inport
  Action Port : ActionPort  ActionPortLabel=if(u1 > 0)
  Out1 : Outport  VectorParamsAs1DForOutWhenUnconnected=off
  wires:
  In1/1 -> Out1/1

== system Control_v8_PID_LLSat/Attitude Controller/Magnetorquer Magnetic Momend Command/Switch Case Action Subsystem4 ==
  In1 : Inport
  Action Port : ActionPort  ActionPortLabel=else
  Out1 : Outport  VectorParamsAs1DForOutWhenUnconnected=off
  wires:
  In1/1 -> Out1/1

== system Control_v8_PID_LLSat/Attitude Controller/PID (nominal command)/Command Magnetic moments computation ==
  note: Moment magnétique de commande M :
      |
      | $M_c = \frac{1}{B²}\vec{B} \wedge\vec{T_P}$
      |
      | Avec Tp couple projeté dans le plan orthogonal à B
      | $T_P=\vec{T}-\frac{1}{B²}(\vec{T}\cdot\vec{B})\vec{B}$
  Command (vect) : Inport  OutDataTypeStr=double
  B_IGRF_body (vect) : Inport  Port=2  OutDataTypeStr=double
  h1 (vect) : Inport  Port=3
  h2 (vect) : Inport  Port=4
  h3 (vect) : Inport  Port=5
  Cross Product : vrlib/Utilities/Cross Product
  Dot Product : DotProduct  OutDataTypeStr=Inherit: Inherit via internal rule
  Global magnetic moment computation : Subsystem
  Mux : Mux  Inputs=3
  Product1 : Product  Inputs=*/
  Reshape : Reshape  OutputDimensionality=Column vector (2-D)
  Reshape1 : Reshape  OutputDimensionality=Column vector (2-D)
  Mag vector command : Outport  VectorParamsAs1DForOutWhenUnconnected=off
  wires:
  B_IGRF_body (vect)/1 -> Reshape1/1  "B_Body"
  Command (vect)/1 -> Reshape/1  "T_Body"
  h1 (vect)/1 -> Global magnetic moment computation/2(In2)
  h2 (vect)/1 -> Global magnetic moment computation/3(In3)
  h3 (vect)/1 -> Global magnetic moment computation/4(In4)
  Global magnetic moment computation/2(magnetic moment 2 (scalar)) -> Mux/2  "magnetic moment 2"
  Global magnetic moment computation/3(magnetic moment 3 (scalar)) -> Mux/3  "magnetic moment 3"
  Global magnetic moment computation/1(magnetic moment 1 (scalar)) -> Mux/1  "magnetic moment 1"
  Mux/1 -> Mag vector command/1
  Reshape1/1 -> Cross Product/2, Dot Product/2, Dot Product/1
  Cross Product/1 -> Product1/1
  Product1/1 -> Global magnetic moment computation/1(In1)  "Mc"
  Dot Product/1 -> Product1/2  "B^2"
  Reshape/1 -> Cross Product/1  "Tp"

== system Control_v8_PID_LLSat/Attitude Controller/PID (nominal command)/Extract Vect ==
  Qr : Inport
  Demux : Demux
  Mux1 : Mux  Inputs=3
  Product : Product
  Reshape : Reshape  OutputDimensionality=Column vector (2-D)
  Sign : Signum
  Qvect : Outport  VectorParamsAs1DForOutWhenUnconnected=off
  wires:
  Demux/2 -> Mux1/1
  Demux/4 -> Mux1/3
  Demux/3 -> Mux1/2
  Demux/1 -> Sign/1
  Qr/1 -> Demux/1
  Mux1/1 -> Product/2
  Product/1 -> Reshape/1
  Sign/1 -> Product/1
  Reshape/1 -> Qvect/1

== system Control_v8_PID_LLSat/Attitude Controller/PID (nominal command)/If Action Subsystem ==
  In1 : Inport
  Action Port : ActionPort  ActionPortLabel=else
  Out1 : Outport  VectorParamsAs1DForOutWhenUnconnected=off
  wires:
  In1/1 -> Out1/1

== system Control_v8_PID_LLSat/Attitude Controller/PID (nominal command)/If Action Subsystem1 ==
  In1 : Inport
  Action Port : ActionPort  ActionPortLabel=if(u1 > 0)
  Out1 : Outport  VectorParamsAs1DForOutWhenUnconnected=off
  wires:
  In1/1 -> Out1/1

== system Control_v8_PID_LLSat/Attitude Controller/PID (nominal command)/If Action Subsystem2 ==
  In1 : Inport
  Action Port : ActionPort  ActionPortLabel=if(u1 > 0.0068)
  Out1 : Outport  VectorParamsAs1DForOutWhenUnconnected=off
  wires:
  In1/1 -> Out1/1

== system Control_v8_PID_LLSat/Attitude Controller/PID (nominal command)/If Action Subsystem3 ==
  In1 : Inport
  Action Port : ActionPort  ActionPortLabel=else
  Out1 : Outport  VectorParamsAs1DForOutWhenUnconnected=off
  wires:
  In1/1 -> Out1/1

== system Control_v8_PID_LLSat/Attitude Controller/PID (nominal command)/RW1 ==
  note: Entrées:
      | - Moment de commande (déjà projeté sur l'axe de la roue...)
      | Sorties:
      | - Omega de commande à appliquer
  Mc (scalar) : Inport
  Discrete-Time Integrator : DiscreteIntegrator  IntegratorMethod=Integration: Trapezoidal  SampleTime=-1  ICPrevOutput=DiscIntNeverNeededParam  ICPrevScaledInput=DiscIntNeverNeededParam
  Divide : Product  Inputs=*/
  Saturation_speed : Saturate  UpperLimit=sat.wheel.max_speed  LowerLimit=- sat.wheel.max_speed
  Torque_sat : Saturate  UpperLimit=sat.wheel.max_torque  LowerLimit=- sat.wheel.max_torque
  Wheel Inertia : Constant  Value=sat.wheel.max_sigma/sat.wheel.max_speed
  Omega_C (scalar) : Outport
  wires:
  Wheel Inertia/1 -> Divide/2
  Divide/1 -> Discrete-Time Integrator/1  "dw/dt"
  Discrete-Time Integrator/1 -> Saturation_speed/1
  Torque_sat/1 -> Divide/1  "Torque (scal)"
  Saturation_speed/1 -> Omega_C (scalar)/1
  Mc (scalar)/1 -> Torque_sat/1

== system Control_v8_PID_LLSat/Attitude Controller/PID (nominal command)/RW2 ==
  note: Entrées:
      | - Moment de commande (déjà projeté sur l'axe de la roue...)
      | Sorties:
      | - Omega de commande à appliquer
  Mc (scalar) : Inport
  Discrete-Time Integrator : DiscreteIntegrator  IntegratorMethod=Integration: Trapezoidal  SampleTime=-1  ICPrevOutput=DiscIntNeverNeededParam  ICPrevScaledInput=DiscIntNeverNeededParam
  Divide : Product  Inputs=*/
  Saturation_speed : Saturate  UpperLimit=sat.wheel.max_speed  LowerLimit=- sat.wheel.max_speed
  Torque_sat : Saturate  UpperLimit=sat.wheel.max_torque  LowerLimit=- sat.wheel.max_torque
  Wheel Inertia : Constant  Value=sat.wheel.max_sigma/sat.wheel.max_speed
  Omega_C (scalar) : Outport
  wires:
  Wheel Inertia/1 -> Divide/2
  Divide/1 -> Discrete-Time Integrator/1  "dw/dt"
  Discrete-Time Integrator/1 -> Saturation_speed/1
  Torque_sat/1 -> Divide/1  "Torque (scal)"
  Saturation_speed/1 -> Omega_C (scalar)/1
  Mc (scalar)/1 -> Torque_sat/1

== system Control_v8_PID_LLSat/Attitude Controller/PID (nominal command)/RW3 ==
  note: Entrées:
      | - Moment de commande (déjà projeté sur l'axe de la roue...)
      | Sorties:
      | - Omega de commande à appliquer
  Mc (scalar) : Inport
  Discrete-Time Integrator : DiscreteIntegrator  IntegratorMethod=Integration: Trapezoidal  SampleTime=-1  ICPrevOutput=DiscIntNeverNeededParam  ICPrevScaledInput=DiscIntNeverNeededParam
  Divide : Product  Inputs=*/
  Saturation_speed : Saturate  UpperLimit=sat.wheel.max_speed  LowerLimit=- sat.wheel.max_speed
  Torque_sat : Saturate  UpperLimit=sat.wheel.max_torque  LowerLimit=- sat.wheel.max_torque
  Wheel Inertia : Constant  Value=sat.wheel.max_sigma/sat.wheel.max_speed
  Omega_C (scalar) : Outport
  wires:
  Wheel Inertia/1 -> Divide/2
  Divide/1 -> Discrete-Time Integrator/1  "dw/dt"
  Discrete-Time Integrator/1 -> Saturation_speed/1
  Torque_sat/1 -> Divide/1  "Torque (scal)"
  Saturation_speed/1 -> Omega_C (scalar)/1
  Mc (scalar)/1 -> Torque_sat/1

== system Control_v8_PID_LLSat/Attitude Controller/PID (nominal command)/RW4  ==
  note: Entrées:
      | - Moment de commande (déjà projeté sur l'axe de la roue...)
      | Sorties:
      | - Omega de commande à appliquer
  Mc (scalar) : Inport
  Discrete-Time Integrator : DiscreteIntegrator  IntegratorMethod=Integration: Trapezoidal  SampleTime=-1  ICPrevOutput=DiscIntNeverNeededParam  ICPrevScaledInput=DiscIntNeverNeededParam
  Divide : Product  Inputs=*/
  Saturation_speed : Saturate  UpperLimit=sat.wheel.max_speed  LowerLimit=- sat.wheel.max_speed
  Torque_sat : Saturate  UpperLimit=sat.wheel.max_torque  LowerLimit=- sat.wheel.max_torque
  Wheel Inertia : Constant  Value=sat.wheel.max_sigma/sat.wheel.max_speed
  Omega_C (scalar) : Outport
  wires:
  Wheel Inertia/1 -> Divide/2
  Divide/1 -> Discrete-Time Integrator/1  "dw/dt"
  Discrete-Time Integrator/1 -> Saturation_speed/1
  Torque_sat/1 -> Divide/1  "Torque (scal)"
  Saturation_speed/1 -> Omega_C (scalar)/1
  Mc (scalar)/1 -> Torque_sat/1

== system Control_v8_PID_LLSat/Attitude Controller/PID (nominal command)/RW5 ==
  note: Entrées:
      | - Moment de commande (déjà projeté sur l'axe de la roue...)
      | Sorties:
      | - Omega de commande à appliquer
  Mc (scalar) : Inport
  Discrete-Time Integrator : DiscreteIntegrator  IntegratorMethod=Integration: Trapezoidal  SampleTime=-1  ICPrevOutput=DiscIntNeverNeededParam  ICPrevScaledInput=DiscIntNeverNeededParam
  Divide : Product  Inputs=*/
  Saturation_speed : Saturate  UpperLimit=sat.wheel.max_speed  LowerLimit=- sat.wheel.max_speed
  Torque_sat : Saturate  UpperLimit=sat.wheel.max_torque  LowerLimit=- sat.wheel.max_torque
  Wheel Inertia : Constant  Value=sat.wheel.max_sigma/sat.wheel.max_speed
  Omega_C (scalar) : Outport
  wires:
  Wheel Inertia/1 -> Divide/2
  Divide/1 -> Discrete-Time Integrator/1  "dw/dt"
  Discrete-Time Integrator/1 -> Saturation_speed/1
  Torque_sat/1 -> Divide/1  "Torque (scal)"
  Saturation_speed/1 -> Omega_C (scalar)/1
  Mc (scalar)/1 -> Torque_sat/1

== system Control_v8_PID_LLSat/Attitude Controller/PID (nominal command)/RW6 ==
  note: Entrées:
      | - Moment de commande (déjà projeté sur l'axe de la roue...)
      | Sorties:
      | - Omega de commande à appliquer
  Mc (scalar) : Inport
  Discrete-Time Integrator : DiscreteIntegrator  IntegratorMethod=Integration: Trapezoidal  SampleTime=-1  ICPrevOutput=DiscIntNeverNeededParam  ICPrevScaledInput=DiscIntNeverNeededParam
  Divide : Product  Inputs=*/
  Saturation_speed : Saturate  UpperLimit=sat.wheel.max_speed  LowerLimit=- sat.wheel.max_speed
  Torque_sat : Saturate  UpperLimit=sat.wheel.max_torque  LowerLimit=- sat.wheel.max_torque
  Wheel Inertia : Constant  Value=sat.wheel.max_sigma/sat.wheel.max_speed
  Omega_C (scalar) : Outport
  wires:
  Wheel Inertia/1 -> Divide/2
  Divide/1 -> Discrete-Time Integrator/1  "dw/dt"
  Discrete-Time Integrator/1 -> Saturation_speed/1
  Torque_sat/1 -> Divide/1  "Torque (scal)"
  Saturation_speed/1 -> Omega_C (scalar)/1
  Mc (scalar)/1 -> Torque_sat/1

== system Control_v8_PID_LLSat/Attitude Controller/Reaction Wheels Speed Command/Switch Case Action Subsystem3 ==
  In1 : Inport
  Action Port : ActionPort  ActionPortLabel=if(u1 > 0)
  Out1 : Outport  VectorParamsAs1DForOutWhenUnconnected=off
  wires:
  In1/1 -> Out1/1

== system Control_v8_PID_LLSat/Attitude Controller/Reaction Wheels Speed Command/Switch Case Action Subsystem4 ==
  In1 : Inport
  Action Port : ActionPort  ActionPortLabel=else
  Out1 : Outport  VectorParamsAs1DForOutWhenUnconnected=off
  wires:
  In1/1 -> Out1/1
